simulink model "BerkLabWork1"  (R2020b)
settings: Solver=VariableStepAuto  StartTime=0.0  StopTime=10.0  RelTol=1e-3
model workspace (MAT data in the model file):
  auto = Simulink.Parameter
  auto.DataType = 'auto'
  auto.Dimensions = [0 0]
settings Model: Creator=90534  LastModifiedBy=User

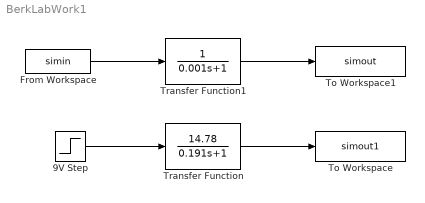
== system BerkLabWork1 ==
  9V Step : Step  Time=0  After=9  SampleTime=0.0001
  From Workspace : FromWorkspace  VariableName=simin
  To Workspace : ToWorkspace  VariableName=simout1  SaveFormat=Timeseries  SampleTime=0.0001
  To Workspace1 : ToWorkspace  VariableName=simout  SaveFormat=Timeseries  SampleTime=0.0001
  Transfer Function : TransferFcn  Numerator=[14.78]  Denominator=[0.191 1]
  Transfer Function1 : TransferFcn  Denominator=[0.001 1]
  wires:
  9V Step/1 -> Transfer Function/1
  Transfer Function/1 -> To Workspace/1
  From Workspace/1 -> Transfer Function1/1
  Transfer Function1/1 -> To Workspace1/1
